simulink model "VL10"  (R2017a)
settings: Solver=FixedStepDiscrete  StartTime=0.0  StopTime=inf  FixedStep=1e-4  RelTol=1e-3
PreLoadFcn:
  | commutationMatrix = load('commutationMatrixFile.mat', '-ascii');
undefined symbols (not defined in the file or in its folder): DiscIntNeverNeededParam
libraries: eltreclib x22, powerlib x21, simulink x1
settings Model: Creator=mayartmal  LastModifiedBy=OspanbekovBK
settings SolverCC: AlgebraicLoopSolver=LineSearch

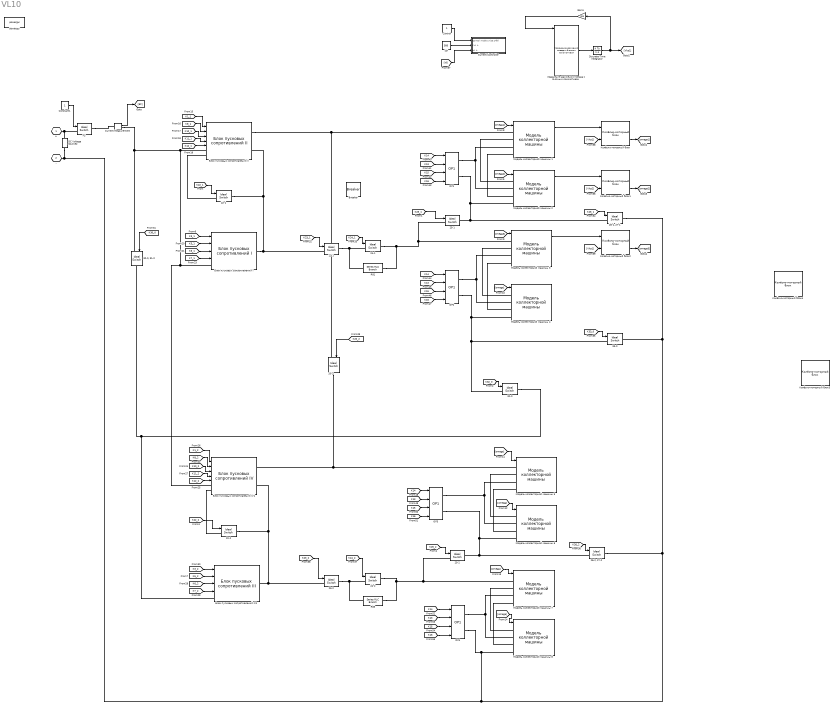
== system VL10 ==
  20-2 : powerlib/Power Electronics/Ideal Switch  Ron=0.001  Lon=0  IC=0  Rs=1e6  Cs=inf  Measurements=off
  22-1 : powerlib/Power Electronics/Ideal Switch  Ron=0.001  Lon=0  IC=0  Rs=1e6  Cs=inf  Measurements=off
  22-2 : powerlib/Power Electronics/Ideal Switch  Ron=0.001  Lon=0  IC=0  Rs=1e6  Cs=inf  Measurements=off
  23-1 : powerlib/Power Electronics/Ideal Switch  Ron=0.001  Lon=0  IC=0  Rs=1e6  Cs=inf  Measurements=off
  23-2 : powerlib/Power Electronics/Ideal Switch  Ron=0.001  Lon=0  IC=0  Rs=1e6  Cs=inf  Measurements=off
  24-1 : powerlib/Power Electronics/Ideal Switch  Ron=0.001  Lon=0  IC=0  Rs=1e6  Cs=inf  Measurements=off
  24-2 : powerlib/Power Electronics/Ideal Switch  Ron=0.001  Lon=0  IC=0  Rs=1e6  Cs=inf  Measurements=off
  25-1 : powerlib/Power Electronics/Ideal Switch  Ron=0.001  Lon=0  IC=0  Rs=1e6  Cs=inf  Measurements=off
  25-2 : powerlib/Power Electronics/Ideal Switch  Ron=0.001  Lon=0  IC=0  Rs=1e6  Cs=inf  Measurements=off
  "26-1, 27-1" : powerlib/Power Electronics/Ideal Switch  Ron=0.001  Lon=0  IC=0  Rs=1e6  Cs=inf  Measurements=off
  "26-2, 27-2" : powerlib/Power Electronics/Ideal Switch  Ron=0.001  Lon=0  IC=0  Rs=1e6  Cs=inf  Measurements=off
  "30-0, 31-0" : powerlib/Power Electronics/Ideal Switch  Ron=0.001  Lon=0  IC=0  Rs=1e6  Cs=inf  Measurements=off
  32-0 : powerlib/Power Electronics/Ideal Switch  Ron=0.001  Lon=0  IC=0  Rs=1e6  Cs=inf  Measurements=off
  33-0 : powerlib/Power Electronics/Ideal Switch  Ron=0.001  Lon=0  IC=0  Rs=1e6  Cs=inf  Measurements=off
  Breaker : powerlib/Elements/Breaker  InitialState=0  SwitchingTimes="[1/60  5/60]"  External=on  BreakerResistance=0.01  SnubberResistance=1e6  SnubberCapacitance=inf  Measurements=None  MoreParameters=on  NoBreakLoop=off
      settings: SourceProductName=Simscape Power Systems
  Constant1 : Constant
  Control : Constant
  Current Controller : Subsystem
  Current Measurement : powerlib/Measurements/Current Measurement  PhasorSimulation=off  OutputType=Complex  PSBequivalent=0
  DC Voltage Source2 : powerlib/Electrical Sources/DC Voltage Source  Amplitude=3000  Measurements=None
  Discrete-Time Integrator : DiscreteIntegrator  InitialConditionSetting=State (most efficient)  SampleTime=-1  ICPrevOutput=DiscIntNeverNeededParam  ICPrevScaledInput=DiscIntNeverNeededParam
  FS : powerlib/Power Electronics/Ideal Switch  Ron=0.001  Lon=0  IC=0  Rs=1e6  Cs=inf  Measurements=off
  Gain1 : Gain  Gain=3.6
  Id* : Constant  Value=500
  OP{1..4} (4 alike) : eltreclib/OP1
      settings: SourceProductName=Electric Traction
  R81 : powerlib/Elements/Series RLC Branch  LConnTagsString=__new0  RConnTagsString=__new0  BranchType=R  Resistance=2.1  Inductance=1e-3  SetiL0=off  InitialCurrent=0  Capacitance=1e-6  Setx0=off  InitialVoltage=0  Measurements=None
  R83 : powerlib/Elements/Series RLC Branch  LConnTagsString=__new0  RConnTagsString=__new0  BranchType=R  Resistance=2.1  Inductance=1e-3  SetiL0=off  InitialCurrent=0  Capacitance=1e-6  Setx0=off  InitialVoltage=0  Measurements=None
  powergui : powerlib/powergui  Priority=1  SimulationMode=Discrete  SampleTime=1e-4  frequency=60  Iterations=50  frequencyindice=0  Pbase=100e6  ErrMax=1e-4  UnitsV=kV  UnitsW=MW  buscounter=0  FunctionMessages=off  echomessages=off  EnableUseOfTLC=off  CurrentSourceSwitches=off  DisableSnubberDevices=off  DisableRonSwitches=off  DisableVfSwitches=off  DisplayEquations=off  SolverType=Tustin/Backward Euler (TBE)  Interpol=off  ExternalGateDelay=off  methode=off  Ts=100  x0status=blocks  SPID=on  SwTol=0  HookPort=off  RestoreLinks=warning  ResistiveCurrentMeasurement=off  Frange=[0:2:500]  Ylog=off  Xlog=on  ShowGrid=off  save=off  variable=ZData  structure=0  ZoomFFT=off  StartTime=0.0  cycles=1  DisplayStyle=1  fundamental=60  FreqAxis=off  MaxFrequency=1000  frequencyindicesteady=1  RmsSteady=1  display=off
  Блок пусковых сопротивлений I : eltreclib/Пусковые сопротивления электровоза ВЛ10/Блок пусковых сопротивлений I
      settings: SourceProductName=Electric Traction
  Блок пусковых сопротивлений II : eltreclib/Пусковые сопротивления электровоза ВЛ10/Блок пусковых сопротивлений II
      settings: SourceProductName=Electric Traction
  Блок пусковых сопротивлений III1 : eltreclib/Пусковые сопротивления электровоза ВЛ10/Блок пусковых сопротивлений III
      settings: SourceProductName=Electric Traction
  Блок пусковых сопротивлений IV1 : eltreclib/Пусковые сопротивления электровоза ВЛ10/Блок пусковых сопротивлений IV
      settings: SourceProductName=Electric Traction
  Колёсно-моторный блок : eltreclib/Колёсно-моторный блок  Db=1.25  mu=3.826
      settings: SourceProductName=Electric Traction
  Колёсно-моторный блок1 : eltreclib/Колёсно-моторный блок  Db=1.25  mu=3.826
      settings: SourceProductName=Electric Traction
  Колёсно-моторный блок2 : eltreclib/Колёсно-моторный блок  Db=1.25  mu=3.826
      settings: SourceProductName=Electric Traction
  Колёсно-моторный блок3 : eltreclib/Колёсно-моторный блок  Db=0  mu=0
  Колёсно-моторный блок4 : eltreclib/Колёсно-моторный блок  Db=0  mu=0
  Модель коллекторной машины {1..8} (8 alike) : eltreclib/Модель коллекторной машины  Rf=0.036  Lf=0.0002  Ra=0.0673  La=0.005  Ce=167.113  Cm=167.113  A=1494  B=6.82
      settings: SourceProductName=Electric Traction
  Уравнение движения поезда c 8-осным локомотивом : eltreclib/Уравнение движения поезда c 8-осным локомотивом  a0=1  a1=0.04  a2=0.0001  P=200  Q=4000
      settings: SourceProductName=Electric Traction
  + : PMIOPort  Tag=PMCPort  Port=1  Side=Left
  - : PMIOPort  Tag=PMCPort  Port=2  Side=Left
  wires:
  [K22_1] -> 22-1/1
  [K25_1] -> 25-1/1
  [K32_0] -> 32-0/1
  [K3_2] -> Блок пусковых сопротивлений III1/1
  Модель коллекторной машины 1/1 -> Колёсно-моторный блок/1
  Gain1/1 -> Уравнение движения поезда c 8-осным локомотивом/1
  Уравнение движения поезда c 8-осным локомотивом/1 -> Discrete-Time Integrator/1
  Discrete-Time Integrator/1 -> [Vkp1], Gain1/1
  [omega1] -> Модель коллекторной машины 1/1
  [omega3] -> Модель коллекторной машины 3/1
  [omega] -> Модель коллекторной машины 4/1
  [omega] -> Модель коллекторной машины 5/1
  [omega] -> Модель коллекторной машины 6/1
  [omega] -> Модель коллекторной машины 7/1
  [omega] -> Модель коллекторной машины 8/1
  [K1_1] -> Блок пусковых сопротивлений II/1
  [K8_1] -> Блок пусковых сопротивлений II/2
  [K10_1] -> Блок пусковых сопротивлений II/3
  [K11_1] -> Блок пусковых сопротивлений II/4
  [K12_1] -> Блок пусковых сопротивлений II/5
  [K3_1] -> Блок пусковых сопротивлений I/1
  [K5_1] -> Блок пусковых сопротивлений I/2
  [K6_1] -> Блок пусковых сопротивлений I/3
  [K7_1] -> Блок пусковых сопротивлений I/4
  [K12_2] -> Блок пусковых сопротивлений IV1/5
  [K1_2] -> Блок пусковых сопротивлений IV1/1
  [K8_2] -> Блок пусковых сопротивлений IV1/2
  [K10_2] -> Блок пусковых сопротивлений IV1/3
  [K11_2] -> Блок пусковых сопротивлений IV1/4
  [K5_2] -> Блок пусковых сопротивлений III1/2
  [K6_2] -> Блок пусковых сопротивлений III1/3
  [K7_2] -> Блок пусковых сопротивлений III1/4
  [K30_0] -> "30-0, 31-0"/1
  [K23_1] -> 23-1/1
  [K24_1] -> 24-1/1
  [K26_1] -> "26-1, 27-1"/1
  [K33_0] -> 33-0/1
  [K26_2] -> "26-2, 27-2"/1
  [K25_2] -> 25-2/1
  [K24_2] -> 24-2/1
  [K23_2] -> 23-2/1
  [K22_2] -> 22-2/1
  [K20_2] -> 20-2/1
  Constant1/1 -> FS/1
  Колёсно-моторный блок/2 -> [omega1]
  [omega2] -> Модель коллекторной машины 2/1
  [K14] -> OP1/1
  [K13] -> OP1/2
  [K15] -> OP1/3
  [K16] -> OP1/4
  [K14] -> OP2/1
  [K13] -> OP2/2
  [K15] -> OP2/3
  [K16] -> OP2/4
  [K14] -> OP3/1
  [K13] -> OP3/2
  [K15] -> OP3/3
  [K16] -> OP3/4
  [K14] -> OP4/1
  [K16] -> OP4/4
  [K15] -> OP4/3
  [K13] -> OP4/2
  Current Measurement/1 -> [EC]
  Control/1 -> Current Controller/1(Control mode 1-rise 2-fall)
  Id*/1 -> Current Controller/2("I*d, A")
  [Id] -> Current Controller/3("Id, A")
  [Vkp1] -> Колёсно-моторный блок/2
  [Vkp2] -> Колёсно-моторный блок1/2
  Колёсно-моторный блок1/2 -> [omega2]
  Модель коллекторной машины 2/1 -> Колёсно-моторный блок1/1
  [Vkp1] -> Колёсно-моторный блок2/2
  Колёсно-моторный блок2/2 -> [omega3]
  Модель коллекторной машины 3/1 -> Колёсно-моторный блок2/1
  connections:
  22-1/LConn1 -- Блок пусковых сопротивлений II/LConn2
  Блок пусковых сопротивлений I/LConn1 -- Current Measurement/RConn1 -- "30-0, 31-0"/LConn1 -- Блок пусковых сопротивлений II/LConn1 -- Блок пусковых сопротивлений IV1/LConn1
  23-1/RConn1 -- R81/LConn1 -- 24-1/LConn1
  OP1/RConn1 -- Модель коллекторной машины 1/LConn3 -- Модель коллекторной машины 2/LConn2
  Блок пусковых сопротивлений II/RConn1 -- Модель коллекторной машины 1/LConn1 -- 20-2/LConn1
  OP1/RConn2 -- Модель коллекторной машины 2/LConn4 -- "26-1, 27-1"/LConn1 -- 25-1/RConn1
  Модель коллекторной машины 2/LConn1 -- Модель коллекторной машины 1/LConn2
  Модель коллекторной машины 2/LConn3 -- Модель коллекторной машины 1/LConn4
  OP2/RConn1 -- Модель коллекторной машины 3/LConn3 -- Модель коллекторной машины 4/LConn2
  OP2/RConn2 -- Модель коллекторной машины 4/LConn4 -- 33-0/LConn1 -- 32-0/LConn1
  Модель коллекторной машины 4/LConn3 -- Модель коллекторной машины 3/LConn4
  Модель коллекторной машины 4/LConn1 -- Модель коллекторной машины 3/LConn2
  22-1/RConn1 -- Блок пусковых сопротивлений II/RConn2 -- Блок пусковых сопротивлений I/RConn1 -- 23-1/LConn1
  24-1/RConn1 -- R81/RConn1 -- Модель коллекторной машины 3/LConn1 -- 25-1/LConn1
  32-0/RConn1 -- "30-0, 31-0"/RConn1 -- Блок пусковых сопротивлений III1/LConn1
  R83/LConn1 -- 23-2/RConn1 -- 24-2/LConn1
  OP3/RConn1 -- Модель коллекторной машины 5/LConn3 -- Модель коллекторной машины 6/LConn2
  Модель коллекторной машины 6/LConn4 -- OP3/RConn2 -- "26-2, 27-2"/LConn1 -- 25-2/RConn1
  OP4/RConn1 -- Модель коллекторной машины 7/LConn3 -- Модель коллекторной машины 8/LConn2
  22-2/RConn1 -- Блок пусковых сопротивлений IV1/RConn2 -- Блок пусковых сопротивлений III1/RConn1 -- 23-2/LConn1
  R83/RConn1 -- 24-2/RConn1 -- Модель коллекторной машины 7/LConn1 -- 25-2/LConn1
  Модель коллекторной машины 6/LConn3 -- Модель коллекторной машины 5/LConn4
  OP4/RConn2 -- Модель коллекторной машины 8/LConn4 -- -/RConn1 -- DC Voltage Source2/LConn1 -- "26-2, 27-2"/RConn1 -- "26-1, 27-1"/RConn1 -- 33-0/RConn1
  Модель коллекторной машины 6/LConn1 -- Модель коллекторной машины 5/LConn2
  Модель коллекторной машины 5/LConn1 -- Блок пусковых сопротивлений IV1/RConn1 -- 20-2/RConn1
  Модель коллекторной машины 8/LConn3 -- Модель коллекторной машины 7/LConn4
  Модель коллекторной машины 8/LConn1 -- Модель коллекторной машины 7/LConn2
  Блок пусковых сопротивлений IV1/LConn2 -- 22-2/LConn1
  +/RConn1 -- FS/LConn1 -- DC Voltage Source2/RConn1
  FS/RConn1 -- Current Measurement/LConn1

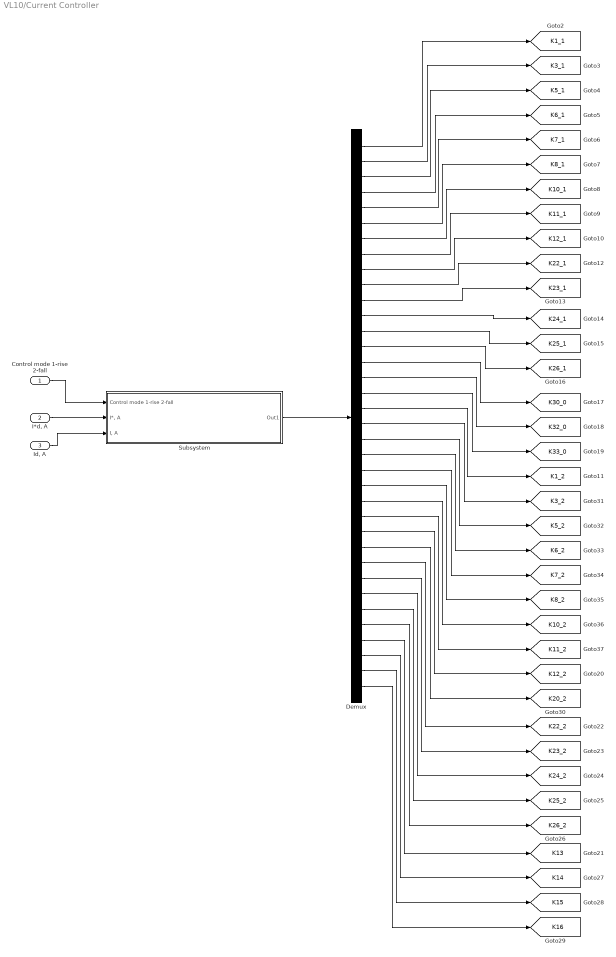
== system VL10/Current Controller ==
  Control mode 1-rise 2-fall : Inport
  "I*d, A" : Inport  Port=2
  "Id, A" : Inport  Port=3
  Demux : Demux  Outputs=36
  Subsystem : Subsystem
  tag scope: K10_1=global, K10_2=global, K11_1=global, K11_2=global, K12_1=global, K12_2=global, K13=global, K14=global, K15=global, K16=global, K1_1=global, K1_2=global, K20_2=global, K22_1=global, K22_2=global, K23_1=global, K23_2=global, K24_1=global, K24_2=global, K25_1=global, K25_2=global, K26_1=global, K26_2=global, K30_0=global, K32_0=global, K33_0=global, K3_1=global, K3_2=global, K5_1=global, K5_2=global, K6_1=global, K6_2=global, K7_1=global, K7_2=global, K8_1=global, K8_2=global
  wires:
  Demux/36 -> [K16]
  Demux/7 -> [K10_1]
  Demux/10 -> [K22_1]
  Demux/8 -> [K11_1]
  Demux/20 -> [K5_2]
  Demux/2 -> [K3_1]
  Demux/11 -> [K23_1]
  Demux/16 -> [K32_0]
  Demux/12 -> [K24_1]
  Demux/19 -> [K3_2]
  Demux/33 -> [K13]
  Demux/22 -> [K7_2]
  Demux/13 -> [K25_1]
  Demux/29 -> [K23_2]
  Demux/34 -> [K14]
  Demux/17 -> [K33_0]
  Demux/30 -> [K24_2]
  Demux/31 -> [K25_2]
  Demux/32 -> [K26_2]
  Demux/15 -> [K30_0]
  "I*d, A"/1 -> Subsystem/2("I*, A")
  Demux/21 -> [K6_2]
  Demux/35 -> [K15]
  Demux/18 -> [K1_2]
  Demux/14 -> [K26_1]
  Control mode 1-rise 2-fall/1 -> Subsystem/1(Control mode 1-rise 2-fall)
  Demux/6 -> [K8_1]
  "Id, A"/1 -> Subsystem/3("I, A")
  Demux/3 -> [K5_1]
  Demux/1 -> [K1_1]
  Demux/23 -> [K8_2]
  Demux/24 -> [K10_2]
  Demux/25 -> [K11_2]
  Demux/5 -> [K7_1]
  Demux/28 -> [K22_2]
  Subsystem/1(Out1) -> Demux/1
  Demux/26 -> [K12_2]
  Demux/27 -> [K20_2]
  Demux/9 -> [K12_1]
  Demux/4 -> [K6_1]

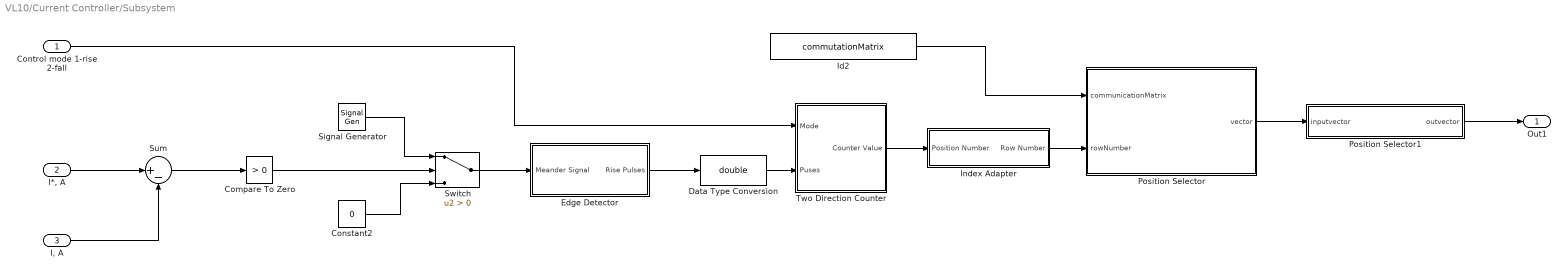
== system VL10/Current Controller/Subsystem ==
  Control mode 1-rise 2-fall : Inport
  "I*, A" : Inport  Port=2
  "I, A" : Inport  Port=3
  Compare To Zero : simulink/Logic and Bit Operations/Compare To Zero  relop=>  OutDataTypeStr=boolean
  Constant2 : Constant  Value=0
  Data Type Conversion : DataTypeConversion  OutDataTypeStr=double
  "Edge Detector " : Subsystem
  Id2 : Constant  Value=commutationMatrix
  Index Adapter : Subsystem
  Position Selector : MATLAB Function  TreatAsAtomicUnit=on
  Position Selector1 : MATLAB Function  TreatAsAtomicUnit=on
  Signal Generator : SignalGenerator  WaveForm=square
  Sum : Sum  Inputs=|+-
  Switch : Switch  Criteria=u2 > Threshold
  Two Direction Counter : Subsystem
  Out1 : Outport
  wires:
  Position Selector/1(vector) -> Position Selector1/1(inputvector)
  "Edge Detector "/1(Rise Pulses) -> Data Type Conversion/1
  Control mode 1-rise 2-fall/1 -> Two Direction Counter/1(Mode)
  Index Adapter/1(Row Number) -> Position Selector/2(rowNumber)
  Id2/1 -> Position Selector/1(communicationMatrix)
  Data Type Conversion/1 -> Two Direction Counter/2(Puses)
  Two Direction Counter/1(Counter Value) -> Index Adapter/1(Position Number)
  Position Selector1/1(outvector) -> Out1/1
  Constant2/1 -> Switch/3
  "I*, A"/1 -> Sum/1
  Sum/1 -> Compare To Zero/1
  Signal Generator/1 -> Switch/1
  Switch/1 -> "Edge Detector "/1(Meander Signal)
  Compare To Zero/1 -> Switch/2
  "I, A"/1 -> Sum/2

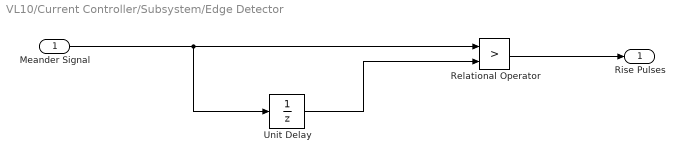
== system VL10/Current Controller/Subsystem/Edge Detector  ==
  Meander Signal : Inport
  Relational Operator : RelationalOperator  Operator=>  OutDataTypeStr=boolean  RndMeth=Simplest
  Unit Delay : UnitDelay  SampleTime=-1
  Rise Pulses : Outport
  wires:
  Unit Delay/1 -> Relational Operator/2
  Meander Signal/1 -> Relational Operator/1, Unit Delay/1
  Relational Operator/1 -> Rise Pulses/1

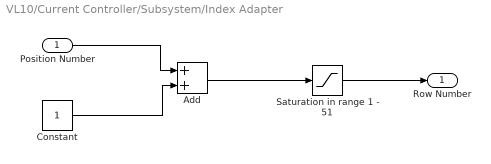
== system VL10/Current Controller/Subsystem/Index Adapter ==
  Position Number : Inport
  Add : Sum
  Constant : Constant
  Saturation in range 1 - 51 : Saturate  UpperLimit=52  LowerLimit=1
  Row Number : Outport
  wires:
  Constant/1 -> Add/2
  Position Number/1 -> Add/1
  Add/1 -> Saturation in range 1 - 51/1
  Saturation in range 1 - 51/1 -> Row Number/1

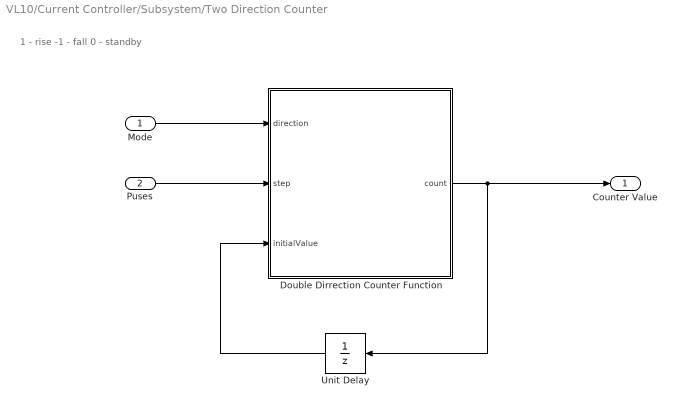
== system VL10/Current Controller/Subsystem/Two Direction Counter ==
  note: 1 - rise
      | -1 - fall
      | 0 - standby
  Mode : Inport
  Puses : Inport  Port=2
  Double Dirrection Counter Function : MATLAB Function  TreatAsAtomicUnit=on
  Unit Delay : UnitDelay  SampleTime=-1
  Counter Value : Outport
  wires:
  Puses/1 -> Double Dirrection Counter Function/2(step)
  Mode/1 -> Double Dirrection Counter Function/1(direction)
  Double Dirrection Counter Function/1(count) -> Counter Value/1, Unit Delay/1
  Unit Delay/1 -> Double Dirrection Counter Function/3(initialValue)

== matlab function VL10/Current Controller/Subsystem/Two Direction Counter/Double Dirrection Counter Function ==
  data: direction input; step input; initialValue input; count output
function count = fcn(direction, step, initialValue)
if direction == 1
    count = initialValue + step;
    if count >= 52
        count = initialValue;
    end
elseif direction == -1
    count = initialValue - step;
    if count < 0
        count = 0;
    end
elseif direction == 0
    count = initialValue;
else
    count = initialValue;
end


% function [count, z]= fcn(direction, step, initialValue)
% z = direction;
% if direction == 1
%     count = initialValue + step;
% else
%     count = initialValue - step;
%     if count < 0
%         count = 0;
%     end
% end
% end

== matlab function VL10/Current Controller/Subsystem/Position Selector ==
  data: communicationMatrix input; vector output; rowNumber input
function vector = fcn(communicationMatrix, rowNumber)
vector = communicationMatrix(rowNumber,:);

== matlab function VL10/Current Controller/Subsystem/Position Selector1 ==
  data: inputvector input; outvector output
function outvector = fcn(inputvector)
outvector = inputvector';
